simulink library "lib_FDM"  (R2019b)
settings: Solver=VariableStepAuto  StartTime=0.0  StopTime=10.0  RelTol=1e-3
values from neighbouring files (symbols this model uses):
  d = config.d_m    [computeTF.m]
undefined symbols (not defined in the file or in its folder): c_b_WGS, c_flat, c_grav, c_rot, c_rsma, Cd0, Cdcl, Cdcl2, Cl0, Cla, Cld, Cma, Cmd, Cmq, Cnb, Cnd, Cnr, Cra, Crd, Crp, Cy0, Cyb, Cyd, dmdt, Earth, HIL_Data, InitThrust, launchPos, me, mf, mp, Sref, tb, TF, theta0, WGS84
libraries: simulink_extras x14, $bdroot x7, simulink x5, lib_Fin_Deflections x3, aerolibasang x2, sharedtransform x1, aerolibtransform2 x1, aerolibbdyn x1, aerolibatmos2 x1, aerolibutil x1, aerolib6dof2 x1
(part 1 of 8)
settings Model: Creator=m.hiepp  LastModifiedBy=Guy
settings DataIOCC: ReturnWorkspaceOutputs=off
settings DebuggingCC: ArithmeticOperatorsInVariantConditions=warning
settings SFSimCC: CustomCodeUndefinedFunction=UseInterfaceOnly

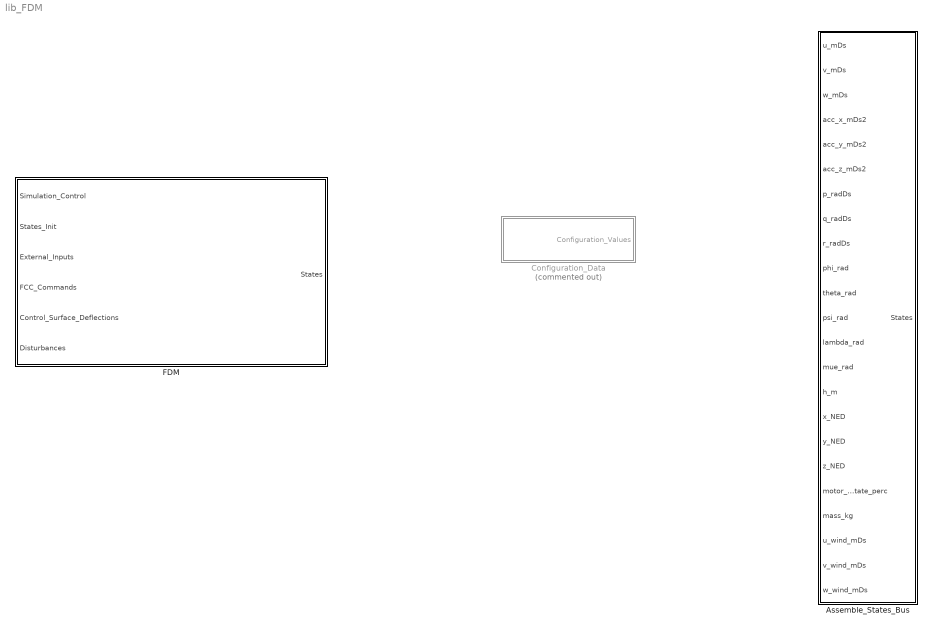
== system lib_FDM ==
  Assemble_States_Bus : Subsystem
  Configuration_Data : Subsystem  Commented=on
  FDM : Subsystem  Variant=on

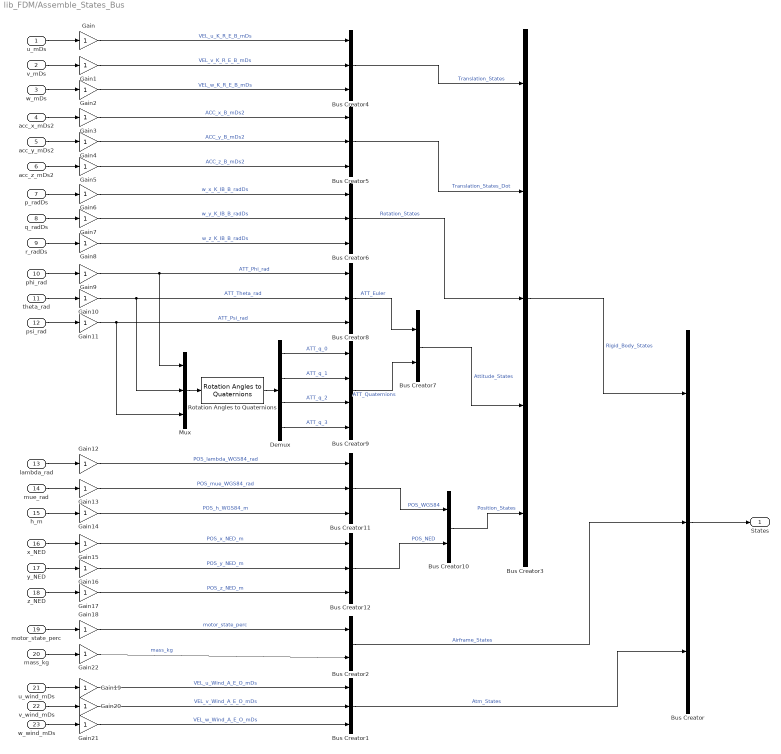
== system lib_FDM/Assemble_States_Bus ==
  u_mDs : Inport
  v_mDs : Inport  Port=2
  w_mDs : Inport  Port=3
  acc_x_mDs2 : Inport  Port=4
  acc_y_mDs2 : Inport  Port=5
  acc_z_mDs2 : Inport  Port=6
  p_radDs : Inport  Port=7
  q_radDs : Inport  Port=8
  r_radDs : Inport  Port=9
  phi_rad : Inport  Port=10
  theta_rad : Inport  Port=11
  psi_rad : Inport  Port=12
  lambda_rad : Inport  Port=13
  mue_rad : Inport  Port=14
  h_m : Inport  Port=15
  x_NED : Inport  Port=16
  y_NED : Inport  Port=17
  z_NED : Inport  Port=18
  motor_state_perc : Inport  Port=19
  mass_kg : Inport  Port=20
  u_wind_mDs : Inport  Port=21
  v_wind_mDs : Inport  Port=22
  w_wind_mDs : Inport  Port=23
  Bus Creator : BusCreator  Inputs=3  OutDataTypeStr=Bus: States_Bus
  Bus Creator1 : BusCreator  Inputs=3  OutDataTypeStr=Bus: Atm_States_Bus
  Bus Creator10 : BusCreator  Inputs=2  OutDataTypeStr=Bus: Position_States_Bus
  Bus Creator11 : BusCreator  Inputs=3  OutDataTypeStr=Bus: POS_WGS84_Bus
  Bus Creator12 : BusCreator  Inputs=3  OutDataTypeStr=Bus: POS_NED_Bus
  Bus Creator2 : BusCreator  Inputs=2  OutDataTypeStr=Bus: Airframe_States_Bus
  Bus Creator3 : BusCreator  Inputs=5  OutDataTypeStr=Bus: Rigid_Body_States_Bus
  Bus Creator4 : BusCreator  Inputs=3  OutDataTypeStr=Bus: Translation_States_Bus
  Bus Creator5 : BusCreator  Inputs=3  OutDataTypeStr=Bus: Translation_States_Dot_Bus
  Bus Creator6 : BusCreator  Inputs=3  OutDataTypeStr=Bus: Rotation_States_Bus
  Bus Creator7 : BusCreator  Inputs=2  OutDataTypeStr=Bus: Attitude_States_Bus
  Bus Creator8 : BusCreator  Inputs=3  OutDataTypeStr=Bus: ATT_Euler_Bus
  Bus Creator9 : BusCreator  Inputs=4  OutDataTypeStr=Bus: ATT_Quaternions_Bus
  Demux : Demux
  Gain{,1..22} (23 alike) : Gain
  Mux : Mux  Inputs=3
  Rotation Angles to Quaternions : sharedtransform/Rotation Angles to Quaternions  rotationOrder=ZYX  aMode=aMode
      settings: SourceProductName=Aerospace Blockset  SourceProductBaseCode=AE
  States : Outport  OutDataTypeStr=Bus: States_Bus  VectorParamsAs1DForOutWhenUnconnected=off
  wires:
  Bus Creator7/1 -> Bus Creator3/4  "Attitude_States"
  Mux/1 -> Rotation Angles to Quaternions/1
  Demux/3 -> Bus Creator9/3  "ATT_q_2"
  Demux/4 -> Bus Creator9/4  "ATT_q_3"
  Demux/1 -> Bus Creator9/1  "ATT_q_0"
  Bus Creator11/1 -> Bus Creator10/1  "POS_WGS84"
  w_mDs/1 -> Gain2/1
  Bus Creator1/1 -> Bus Creator/3  "Atm_States"
  Bus Creator9/1 -> Bus Creator7/2  "ATT_Quaternions"
  acc_x_mDs2/1 -> Gain3/1
  Bus Creator12/1 -> Bus Creator10/2  "POS_NED"
  Demux/2 -> Bus Creator9/2  "ATT_q_1"
  Bus Creator10/1 -> Bus Creator3/5  "Position_States"
  acc_z_mDs2/1 -> Gain5/1
  phi_rad/1 -> Gain9/1
  z_NED/1 -> Gain17/1
  Bus Creator2/1 -> Bus Creator/2  "Airframe_States"
  Bus Creator8/1 -> Bus Creator7/1  "ATT_Euler"
  w_wind_mDs/1 -> Gain21/1
  Bus Creator3/1 -> Bus Creator/1  "Rigid_Body_States"
  u_wind_mDs/1 -> Gain19/1
  Bus Creator4/1 -> Bus Creator3/1  "Translation_States"
  mue_rad/1 -> Gain13/1
  y_NED/1 -> Gain16/1
  Bus Creator6/1 -> Bus Creator3/3  "Rotation_States"
  Bus Creator5/1 -> Bus Creator3/2  "Translation_States_Dot"
  Rotation Angles to Quaternions/1 -> Demux/1
  x_NED/1 -> Gain15/1
  Bus Creator/1 -> States/1
  h_m/1 -> Gain14/1
  u_mDs/1 -> Gain/1
  lambda_rad/1 -> Gain12/1
  v_mDs/1 -> Gain1/1
  v_wind_mDs/1 -> Gain20/1
  motor_state_perc/1 -> Gain18/1
  psi_rad/1 -> Gain11/1
  theta_rad/1 -> Gain10/1
  r_radDs/1 -> Gain8/1
  p_radDs/1 -> Gain6/1
  q_radDs/1 -> Gain7/1
  acc_y_mDs2/1 -> Gain4/1
  Gain20/1 -> Bus Creator1/2  "VEL_v_Wind_A_E_O_mDs"
  Gain21/1 -> Bus Creator1/3  "VEL_w_Wind_A_E_O_mDs"
  Gain19/1 -> Bus Creator1/1  "VEL_u_Wind_A_E_O_mDs"
  Gain18/1 -> Bus Creator2/1  "motor_state_perc"
  Gain17/1 -> Bus Creator12/3  "POS_z_NED_m"
  Gain16/1 -> Bus Creator12/2  "POS_y_NED_m"
  Gain15/1 -> Bus Creator12/1  "POS_x_NED_m"
  Gain14/1 -> Bus Creator11/3  "POS_h_WGS84_m"
  Gain13/1 -> Bus Creator11/2  "POS_mue_WGS84_rad"
  Gain12/1 -> Bus Creator11/1  "POS_lambda_WGS84_rad"
  Gain11/1 -> Bus Creator8/3, Mux/3  "ATT_Psi_rad"
  Gain10/1 -> Bus Creator8/2, Mux/2  "ATT_Theta_rad"
  Gain9/1 -> Bus Creator8/1, Mux/1  "ATT_Phi_rad"
  Gain8/1 -> Bus Creator6/3  "w_z_K_IB_B_radDs"
  Gain7/1 -> Bus Creator6/2  "w_y_K_IB_B_radDs"
  Gain6/1 -> Bus Creator6/1  "w_x_K_IB_B_radDs"
  Gain5/1 -> Bus Creator5/3  "ACC_z_B_mDs2"
  Gain4/1 -> Bus Creator5/2  "ACC_y_B_mDs2"
  Gain3/1 -> Bus Creator5/1  "ACC_x_B_mDs2"
  Gain2/1 -> Bus Creator4/3  "VEL_w_K_R_E_B_mDs"
  Gain1/1 -> Bus Creator4/2  "VEL_v_K_R_E_B_mDs"
  Gain/1 -> Bus Creator4/1  "VEL_u_K_R_E_B_mDs"
  Gain22/1 -> Bus Creator2/2  "mass_kg"
  mass_kg/1 -> Gain22/1

== system lib_FDM/Configuration_Data ==
  Bus Creator : BusCreator  Inputs=10  OutDataTypeStr=Bus: Configuration_Values_Bus
  Constant : Constant  Value=HIL_Data.Configuration_Data.param1
  Configuration_Values : Outport  OutDataTypeStr=Bus: Configuration_Values_Bus  VectorParamsAs1DForOutWhenUnconnected=off
  wires:
  Constant/1 -> Bus Creator/1  "param1"
  Bus Creator/1 -> Configuration_Values/1

== system lib_FDM/FDM ==
  Simulation_Control : Inport  OutDataTypeStr=Bus: Simulation_Ctrl_Bus
  States_Init : Inport  Port=2  OutDataTypeStr=Bus: States_Bus
  External_Inputs : Inport  Port=3  OutDataTypeStr=Bus: External_Inputs_Bus
  FCC_Commands : Inport  Port=4  OutDataTypeStr=Bus: FCC_Commands_Bus
  Control_Surface_Deflections : Inport  Port=5  OutDataTypeStr=Bus: Control_Surface_Deflections_Bus
  Disturbances : Inport  Port=6  OutDataTypeStr=Bus: Disturbances_Bus
  FDM_Basic : Subsystem  VariantControl=VSS_FDM_BASIC  mask{FDM=HIL_Data.FDM, Basic=HIL_Data.FDM.Basic}
      mask prompts: FDM "FDM Data"; Basic "FDM Basic Data"
  FDM_Linear : Subsystem  VariantControl=VSS_FDM_LIN  mask{FDM=HIL_Data.FDM, Lin=HIL_Data.FDM.Lin, TF=HIL_Data.FDM.Lin.TF}
      mask prompts: FDM "FDM Data"; Lin "FDM Lin Data"; TF "Transfer Functions"
  FDM_Sophisticated : Subsystem  VariantControl=VSS_FDM_SOPH
  FDM_Student : Subsystem  VariantControl=VSS_FDM_STUD
  States : Outport  OutDataTypeStr=Bus: States_Bus  VectorParamsAs1DForOutWhenUnconnected=off

== system lib_FDM/FDM/FDM_Basic ==
  note: further commands??
  Simulation_Control : Inport  OutDataTypeStr=Bus: Simulation_Ctrl_Bus
  States_Init : Inport  Port=2  OutDataTypeStr=Bus: States_Bus
  External_Inputs : Inport  Port=3  OutDataTypeStr=Bus: External_Inputs_Bus
  FCC_Commands : Inport  Port=4  OutDataTypeStr=Bus: FCC_Commands_Bus
  Control_Surface_Deflections : Inport  Port=5  OutDataTypeStr=Bus: Control_Surface_Deflections_Bus
  Disturbances : Inport  Port=6  OutDataTypeStr=Bus: FCC_Commands_Bus
  Assemble_States_Bus : $bdroot/Assemble_States_Bus  SystemSampleTime=-1  Latency=0  AutoFrameSizeCalculation=off
  Bus Selector : BusSelector  OutputSignals=Translation_States.VEL_u_K_R_E_B_mDs,Translation_States.VEL_v_K_R_E_B_mDs,Translation_States.VEL_w_K_R_E_B_mDs
  Bus Selector1 : BusSelector  OutputSignals=Translation_States_Dot.ACC_x_B_mDs2,Translation_States_Dot.ACC_y_B_mDs2,Translation_States_Dot.ACC_z_B_mDs2
  Bus Selector2 : BusSelector  OutputSignals=Attitude_States.ATT_Phi_rad,Attitude_States.ATT_Theta_rad,Attitude_States.ATT_Psi_rad,Position_States.POS_WGS84.POS_lambda_ WGS84_rad,Position_States.POS_WGS84.POS_mue_ WGS84_rad,Position_States.POS_WGS84.POS_h_ WGS84_m,Position_States.POS_NED.POS_x_NED_m,Position_States.POS_NED.POS_y_NED_m,Position_States.POS_NED.POS_z_NED_m,Airframe_States.motor_state_perc,Airframe_States.mass_kg
  Bus Selector3 : BusSelector  OutputSignals=p_B_radDs,q_B_radDs,r_B_radDs
  Configuration_Data : $bdroot/Configuration_Data  Commented=on  SystemSampleTime=-1  Latency=0  AutoFrameSizeCalculation=off
  Constant : Constant  Value=-1
  Constant1 : Constant  Value=-1
  Constant2 : Constant  Value=-1
  Flight_State : Subsystem
  Motion_Kinematics : Subsystem
  State_Integration : Subsystem
  Terminator{,1,4..8} (7 alike) : Terminator
  States : Outport  OutDataTypeStr=Bus: States_Bus  VectorParamsAs1DForOutWhenUnconnected=off
  wires:
  Assemble_States_Bus/1 -> States/1
  FCC_Commands/1 -> Terminator/1
  Flight_State/1(vel_mDs) -> Terminator4/1
  Flight_State/4(mach) -> Terminator7/1
  Flight_State/5(q_kgDms2) -> Terminator8/1
  Flight_State/3(rho_kgDm3) -> Terminator6/1
  Flight_State/2(altitude_m) -> Terminator5/1
  State_Integration/1("FDM_States ") -> Motion_Kinematics/4(FDM_States)
  Motion_Kinematics/3(FDM_States_Dot) -> Bus Selector1/1, State_Integration/1(FDM_States_Dot)
  External_Inputs/1 -> Motion_Kinematics/2(External_Inputs)
  Simulation_Control/1 -> Motion_Kinematics/1(Simulation_Control), State_Integration/2(Simulation_Control)
  Control_Surface_Deflections/1 -> Motion_Kinematics/3(Control_Surface_Deflections)
  States_Init/1 -> State_Integration/3(States_Init)
  Motion_Kinematics/1(FDM_states) -> Bus Selector/1, Bus Selector2/1
  Bus Selector1/3 -> Assemble_States_Bus/6  "<ACC_z_B_mDs2>"
  Bus Selector1/2 -> Assemble_States_Bus/5  "<ACC_y_B_mDs2>"
  Bus Selector1/1 -> Assemble_States_Bus/4  "<ACC_x_B_mDs2>"
  Bus Selector/1 -> Assemble_States_Bus/1  "<VEL_u_K_R_E_B_mDs>"
  Bus Selector/2 -> Assemble_States_Bus/2  "<VEL_v_K_R_E_B_mDs>"
  Bus Selector/3 -> Assemble_States_Bus/3  "<VEL_w_K_R_E_B_mDs>"
  Bus Selector2/1 -> Assemble_States_Bus/10  "<ATT_Phi_rad>"
  Bus Selector2/2 -> Assemble_States_Bus/11  "<ATT_Theta_rad>"
  Bus Selector2/3 -> Assemble_States_Bus/12  "<ATT_Psi_rad>"
  Bus Selector2/4 -> Assemble_States_Bus/13  "<POS_lambda_ WGS84_rad>"
  Bus Selector2/5 -> Assemble_States_Bus/14  "<POS_mue_ WGS84_rad>"
  Bus Selector2/6 -> Assemble_States_Bus/15  "<POS_h_ WGS84_m>"
  Bus Selector2/7 -> Assemble_States_Bus/16  "<POS_x_NED_m>"
  Bus Selector2/8 -> Assemble_States_Bus/17  "<POS_y_NED_m>"
  Bus Selector2/9 -> Assemble_States_Bus/18  "<POS_z_NED_m>"
  Bus Selector2/10 -> Assemble_States_Bus/19  "<motor_state_perc>"
  Bus Selector2/11 -> Assemble_States_Bus/20  "<mass_kg>"
  Constant/1 -> Assemble_States_Bus/23
  Constant2/1 -> Assemble_States_Bus/21
  Constant1/1 -> Assemble_States_Bus/22
  Motion_Kinematics/2(FDM_Rot_Body) -> Bus Selector3/1
  Bus Selector3/1 -> Assemble_States_Bus/7  "<p_B_radDs>"
  Bus Selector3/2 -> Assemble_States_Bus/8  "<q_B_radDs>"
  Bus Selector3/3 -> Assemble_States_Bus/9  "<r_B_radDs>"
  Disturbances/1 -> Terminator1/1

== system lib_FDM/FDM/FDM_Linear ==
  note: further commands??
  Simulation_Control : Inport  OutDataTypeStr=Bus: Simulation_Ctrl_Bus
  States_Init : Inport  Port=2  OutDataTypeStr=Bus: States_Bus
  External_Inputs : Inport  Port=3  OutDataTypeStr=Bus: External_Inputs_Bus
  FCC_Commands : Inport  Port=4  OutDataTypeStr=Bus: FCC_Commands_Bus
  Control_Surface_Deflections : Inport  Port=5  OutDataTypeStr=Bus: Control_Surface_Deflections_Bus
  Disturbances : Inport  Port=6  OutDataTypeStr=Bus: FCC_Commands_Bus
  Assemble_States_Bus : $bdroot/Assemble_States_Bus  SystemSampleTime=-1  Latency=0  AutoFrameSizeCalculation=off
  Bus Selector : BusSelector  OutputSignals=Translation_States.VEL_u_K_R_E_B_mDs,Translation_States.VEL_v_K_R_E_B_mDs,Translation_States.VEL_w_K_R_E_B_mDs
  Bus Selector1 : BusSelector  OutputSignals=Translation_States_Dot.ACC_x_B_mDs2,Translation_States_Dot.ACC_y_B_mDs2,Translation_States_Dot.ACC_z_B_mDs2
  Bus Selector2 : BusSelector  OutputSignals=Attitude_States.ATT_Phi_rad,Attitude_States.ATT_Theta_rad,Attitude_States.ATT_Psi_rad,Position_States.POS_WGS84.POS_lambda_ WGS84_rad,Position_States.POS_WGS84.POS_mue_ WGS84_rad,Position_States.POS_WGS84.POS_h_ WGS84_m,Position_States.POS_NED.POS_x_NED_m,Position_States.POS_NED.POS_y_NED_m,Position_States.POS_NED.POS_z_NED_m,Airframe_States.motor_state_perc,Airframe_States.mass_kg
  Bus Selector3 : BusSelector  OutputSignals=p_B_radDs,q_B_radDs,r_B_radDs
  Configuration_Data : $bdroot/Configuration_Data  Commented=on  SystemSampleTime=-1  Latency=0  AutoFrameSizeCalculation=off
  Constant : Constant  Value=-1
  Constant1 : Constant  Value=-1
  Constant2 : Constant  Value=-1
  Flight_State : Subsystem
  Motion_Kinematics : Subsystem
  State_Integration : Subsystem
  Terminator{,1,4..8} (7 alike) : Terminator
  States : Outport  OutDataTypeStr=Bus: States_Bus  VectorParamsAs1DForOutWhenUnconnected=off
  wires:
  Assemble_States_Bus/1 -> States/1
  FCC_Commands/1 -> Terminator/1
  Flight_State/1(vel_mDs) -> Terminator4/1
  Flight_State/4(mach) -> Terminator7/1
  Flight_State/5(q_kgDms2) -> Terminator8/1
  Flight_State/3(rho_kgDm3) -> Terminator6/1
  Flight_State/2(altitude_m) -> Terminator5/1
  State_Integration/1("FDM_States ") -> Motion_Kinematics/4(FDM_States)
  Motion_Kinematics/3(FDM_States_Dot) -> Bus Selector1/1, State_Integration/1(FDM_States_Dot)
  External_Inputs/1 -> Motion_Kinematics/2(External_Inputs)
  Simulation_Control/1 -> Motion_Kinematics/1(Simulation_Control), State_Integration/2(Simulation_Control)
  Control_Surface_Deflections/1 -> Motion_Kinematics/3(Control_Surface_Deflections)
  States_Init/1 -> State_Integration/3(States_Init)
  Motion_Kinematics/1(FDM_states) -> Bus Selector/1, Bus Selector2/1
  Bus Selector1/3 -> Assemble_States_Bus/6  "<ACC_z_B_mDs2>"
  Bus Selector1/2 -> Assemble_States_Bus/5  "<ACC_y_B_mDs2>"
  Bus Selector1/1 -> Assemble_States_Bus/4  "<ACC_x_B_mDs2>"
  Bus Selector/1 -> Assemble_States_Bus/1  "<VEL_u_K_R_E_B_mDs>"
  Bus Selector/2 -> Assemble_States_Bus/2  "<VEL_v_K_R_E_B_mDs>"
  Bus Selector/3 -> Assemble_States_Bus/3  "<VEL_w_K_R_E_B_mDs>"
  Bus Selector2/1 -> Assemble_States_Bus/10  "<ATT_Phi_rad>"
  Bus Selector2/2 -> Assemble_States_Bus/11  "<ATT_Theta_rad>"
  Bus Selector2/3 -> Assemble_States_Bus/12  "<ATT_Psi_rad>"
  Bus Selector2/4 -> Assemble_States_Bus/13  "<POS_lambda_ WGS84_rad>"
  Bus Selector2/5 -> Assemble_States_Bus/14  "<POS_mue_ WGS84_rad>"
  Bus Selector2/6 -> Assemble_States_Bus/15  "<POS_h_ WGS84_m>"
  Bus Selector2/7 -> Assemble_States_Bus/16  "<POS_x_NED_m>"
  Bus Selector2/8 -> Assemble_States_Bus/17  "<POS_y_NED_m>"
  Bus Selector2/9 -> Assemble_States_Bus/18  "<POS_z_NED_m>"
  Bus Selector2/10 -> Assemble_States_Bus/19  "<motor_state_perc>"
  Bus Selector2/11 -> Assemble_States_Bus/20  "<mass_kg>"
  Constant/1 -> Assemble_States_Bus/23
  Constant2/1 -> Assemble_States_Bus/21
  Constant1/1 -> Assemble_States_Bus/22
  Motion_Kinematics/2(FDM_Rot_Body) -> Bus Selector3/1
  Bus Selector3/1 -> Assemble_States_Bus/7  "<p_B_radDs>"
  Bus Selector3/2 -> Assemble_States_Bus/8  "<q_B_radDs>"
  Bus Selector3/3 -> Assemble_States_Bus/9  "<r_B_radDs>"
  Disturbances/1 -> Terminator1/1

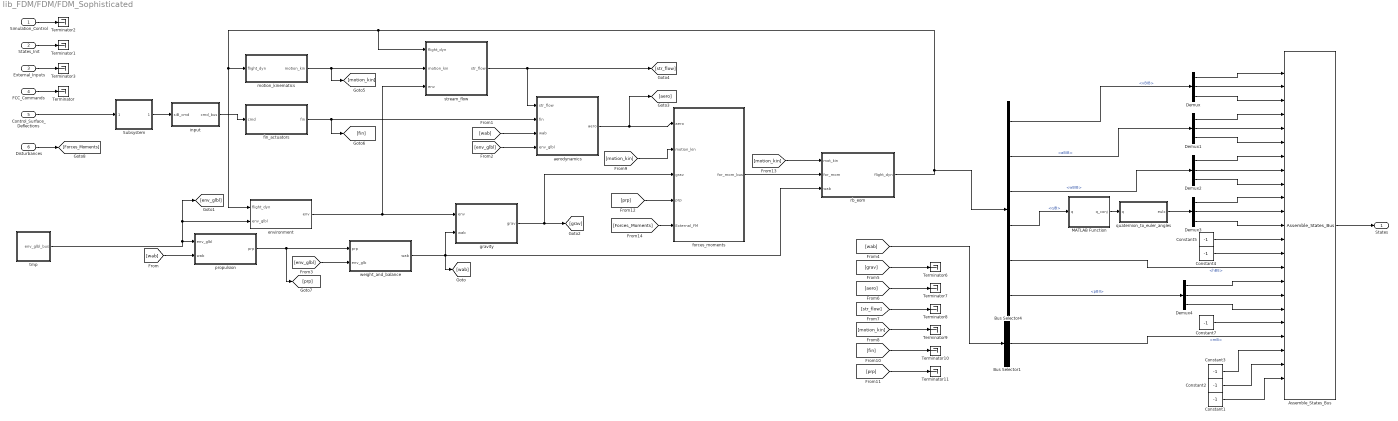
== system lib_FDM/FDM/FDM_Sophisticated ==
  Simulation_Control : Inport  OutDataTypeStr=Bus: Simulation_Ctrl_Bus
  States_Init : Inport  Port=2  OutDataTypeStr=Bus: States_Bus
  External_Inputs : Inport  Port=3  OutDataTypeStr=Bus: External_Inputs_Bus
  FCC_Commands : Inport  Port=4  OutDataTypeStr=Bus: FCC_Commands_Bus
  Control_Surface_Deflections : Inport  Port=5  OutDataTypeStr=Bus: Control_Surface_Deflections_Bus
  Disturbances : Inport  Port=6
  Assemble_States_Bus : $bdroot/Assemble_States_Bus  SystemSampleTime=-1  Latency=0  AutoFrameSizeCalculation=off
  Bus Selector1 : BusSelector  OutputSignals=mB
  Bus Selector4 : BusSelector  OutputSignals=vBIB,aBIB,wBIB,qIB,hBE,pBII
  Constant{1..5,7} (6 alike) : Constant  Value=-1
  Demux{,1..4} (5 alike) : Demux  Outputs=3
  MATLAB Function : MATLAB Function  TreatAsAtomicUnit=on
  Subsystem : Subsystem
  Terminator{,1..3,6..11} (10 alike) : Terminator
  aerodynamics : Subsystem
  environment : Subsystem
  fin_actuators : Subsystem
  forces_moments : Subsystem
  gravity : Subsystem
  input : Subsystem
  motion_kinematics : Subsystem
  propulsion : Subsystem
  quaternion_to_euler_angles : Subsystem
      mask help: transforms quaternions to Euler angles (roll, pitch, yaw)
      mask Help:
      | Name:
      | 
      |     quaternion_to_euler_angles
      | 
      | Description:
      | 
      |     This block implements the transformation of a quaternion into the
      |     corresponding Euler angles (zyx-sequence, roll, pitch, yaw).
      | 
      | Inputs  [size] [data type] [unit]:
      | 
      |     quaternion  [4] [double] [-]
      | 
      | Outputs  [size] [data type] [unit]:
      | 
      |     roll angle phi  [1] [double] [rad]
      |     pitch angle theta  [1] [double] [rad]
      |     yaw angle psi  [1] [double] [rad]
      mask Display:
      | %disp (' q --> (Phi,Theta,Psi) [rad]')
      | disp('q \rightarrow eu(\Phi;\Theta;\Psi)','texmode','on')
  rb_eom : Subsystem
  stream_flow : Subsystem
  tmp : Subsystem
  weight_and_balance : Subsystem
  States : Outport  OutDataTypeStr=Bus: States_Bus  VectorParamsAs1DForOutWhenUnconnected=off
  wires:
  environment/1(env) -> stream_flow/3(env), gravity/1(env)
  motion_kinematics/1(motion_kin) -> [motion_kin], stream_flow/2(motion_kin)
  [wab] -> aerodynamics/3(wab)
  [env_glbl] -> weight_and_balance/2(env_glb)
  fin_actuators/1(fin) -> aerodynamics/2(fin), [fin]
  propulsion/1(prp) -> [prp], weight_and_balance/1(prp)
  forces_moments/1(for_mom_bus) -> rb_eom/2(for_mom)
  aerodynamics/1(aero) -> [aero], forces_moments/1(aero)
  tmp/1(env_glbl_bus) -> environment/2(env_glbl), [env_glbl], propulsion/1(env_glbl)
  [aero] -> Terminator7/1
  [motion_kin] -> forces_moments/2(motion_kin)
  [motion_kin] -> Terminator9/1
  gravity/1(grav) -> forces_moments/3(grav), [grav]
  [motion_kin] -> rb_eom/1(mot_kin)
  [fin] -> Terminator10/1
  [str_flow] -> Terminator8/1
  [wab] -> Bus Selector1/1
  stream_flow/1(str_flow) -> [str_flow], aerodynamics/1(str_flow)
  weight_and_balance/1(wab) -> gravity/2(wab), rb_eom/3(wab), [wab]
  rb_eom/1(flight_dyn) -> motion_kinematics/1(flight_dyn), environment/1(flight_dyn), stream_flow/1(flight_dyn), Bus Selector4/1
  [env_glbl] -> aerodynamics/4(env_glbl)
  input/1(cmd_bus) -> fin_actuators/1(cmd)
  [prp] -> Terminator11/1
  [grav] -> Terminator6/1
  [prp] -> forces_moments/4(prp)
  [wab] -> propulsion/2(wab)
  FCC_Commands/1 -> Terminator/1
  States_Init/1 -> Terminator1/1
  Simulation_Control/1 -> Terminator2/1
  Demux2/1 -> Assemble_States_Bus/7
  Demux2/3 -> Assemble_States_Bus/9
  Demux2/2 -> Assemble_States_Bus/8
  Demux4/3 -> Assemble_States_Bus/18
  Demux4/1 -> Assemble_States_Bus/16
  Constant2/1 -> Assemble_States_Bus/22
  Assemble_States_Bus/1 -> States/1
  Demux3/1 -> Assemble_States_Bus/10
  Constant1/1 -> Assemble_States_Bus/23
  Constant7/1 -> Assemble_States_Bus/19
  Constant4/1 -> Assemble_States_Bus/14
  Constant5/1 -> Assemble_States_Bus/13
  Demux/2 -> Assemble_States_Bus/2
  Demux3/3 -> Assemble_States_Bus/12
  Demux1/1 -> Assemble_States_Bus/4
  Demux/1 -> Assemble_States_Bus/1
  Demux/3 -> Assemble_States_Bus/3
  Constant3/1 -> Assemble_States_Bus/21
  Demux1/2 -> Assemble_States_Bus/5
  Demux1/3 -> Assemble_States_Bus/6
  Demux4/2 -> Assemble_States_Bus/17
  Bus Selector4/1 -> Demux/1  "<vBIB>"
  Bus Selector4/2 -> Demux1/1  "<aBIB>"
  Bus Selector4/3 -> Demux2/1  "<wBIB>"
  Bus Selector4/4 -> MATLAB Function/1(q)  "<qIB>"
  MATLAB Function/1(q_conj) -> quaternion_to_euler_angles/1(q)
  quaternion_to_euler_angles/1(eulx) -> Demux3/1
  Demux3/2 -> Assemble_States_Bus/11
  Bus Selector4/6 -> Demux4/1  "<pBII>"
  Bus Selector4/5 -> Assemble_States_Bus/15  "<hBE>"
  External_Inputs/1 -> Terminator3/1
  [Forces_Moments] -> forces_moments/5(External_FM)
  Disturbances/1 -> [Forces_Moments]
  Bus Selector1/1 -> Assemble_States_Bus/20  "<mB>"
  Control_Surface_Deflections/1 -> Subsystem/1(Servo Deflections)
  Subsystem/1(siB_cmd) -> input/1(siB_cmd)

== system lib_FDM/FDM/FDM_Student ==
  note: TBD!
  note: TBD
  note: TBD: insert propulsion
  note: TBD!
  note: TBD!
  note: TBD!
  Simulation_Control : Inport  OutDataTypeStr=Bus: Simulation_Ctrl_Bus
  States_Init : Inport  Port=2  OutDataTypeStr=Bus: States_Bus
  External_Inputs : Inport  Port=3  OutDataTypeStr=Bus: External_Inputs_Bus
  FCC_Commands : Inport  Port=4  OutDataTypeStr=Bus: FCC_Commands_Bus
  Control_Surface_Deflections : Inport  Port=5  OutDataTypeStr=Bus: Control_Surface_Deflections_Bus
  Aerodynamics : Subsystem
  Assemble_States_Bus : $bdroot/Assemble_States_Bus  SystemSampleTime=-1  Latency=0  AutoFrameSizeCalculation=off
  Configuration_Data : $bdroot/Configuration_Data  Commented=on  SystemSampleTime=-1  Latency=0  AutoFrameSizeCalculation=off
  Demux{,1..5} (6 alike) : Demux  Outputs=3
  Global Calculations : Subsystem
  MATLAB Function : MATLAB Function  TreatAsAtomicUnit=on
  MATLAB Function1 : MATLAB Function  TreatAsAtomicUnit=on
  Memory : Memory
  Reverse Fin Deflection : lib_Fin_Deflections/Reverse Fin Deflection  Control_Surfaces=HIL_Data.Control_Surfaces
  Selector : Selector  InputPortWidth=3  IndexOptions=Index vector (dialog)  Indices=[1]  OutputSizes=1
  Simple Variable Mass 6DOF ECEF (Quaternion) : aerolib6dof2/6DOF ECEF (Quaternion)  units=Metric (MKS)  mtype=Simple Variable  xg_0=[launchPos(1) launchPos(2) launchPos(3)]  Vm_0=[0 0 0]  eul_0=[0 theta0 0]  pm_0=[0 0 0]  mass_0=mf  mass_e=me  mass_f=mf  inertia=inertia  inertia_e=Ie  inertia_f=If  vre_flag=off  abi_flag=on  ptype=Earth (WGS84)  R=6378137  F=1/298.257223563  w_E=7292115e-11  angle_in=Internal  LG0=0  quat_statename=''  pm_statename=''  Vm_statename=''  posECEF_statename=''  posECI_statename=''  LG_statename=''  mass_statename=''
      settings: SourceProductName=Aerospace Blockset  SourceProductBaseCode=AE
  TBD : Constant  Value=-1
  TBD1 : Constant  Value=-1
  Terminator{,1..14} (15 alike) : Terminator
  Transpose : Math  Operator=transpose  SaturateOnIntegerOverflow=on
  States : Outport  OutDataTypeStr=Bus: States_Bus  VectorParamsAs1DForOutWhenUnconnected=off
  wires:
  Aerodynamics/2("[Mxb Myb Mzb]") -> Simple Variable Mass 6DOF ECEF (Quaternion)/2
  [dmdt] -> Simple Variable Mass 6DOF ECEF (Quaternion)/3
  Aerodynamics/1("[Fxb Fyb Fzb]") -> Simple Variable Mass 6DOF ECEF (Quaternion)/1
  Assemble_States_Bus/1 -> States/1
  Reverse Fin Deflection/1 -> Aerodynamics/3(delta R)  "delta_r"
  Reverse Fin Deflection/2 -> Aerodynamics/2(delta P)  "delta_p"
  Reverse Fin Deflection/3 -> Aerodynamics/1("delta Y ")  "delta_y"
  Control_Surface_Deflections/1 -> Reverse Fin Deflection/2
  Simple Variable Mass 6DOF ECEF (Quaternion)/1 -> MATLAB Function/2(VelECEF), Terminator/1
  Simple Variable Mass 6DOF ECEF (Quaternion)/2 -> Terminator1/1, MATLAB Function/3(PosECEF)
  Demux/1 -> Assemble_States_Bus/13
  Demux/2 -> Assemble_States_Bus/14
  Demux/3 -> Assemble_States_Bus/15
  Simple Variable Mass 6DOF ECEF (Quaternion)/3 -> Demux/1
  Demux1/3 -> Assemble_States_Bus/12
  Demux1/2 -> Assemble_States_Bus/11
  Demux1/1 -> Assemble_States_Bus/10
  Simple Variable Mass 6DOF ECEF (Quaternion)/4 -> Demux1/1, Selector/1
  Simple Variable Mass 6DOF ECEF (Quaternion)/5 -> Terminator2/1
  Simple Variable Mass 6DOF ECEF (Quaternion)/6 -> Transpose/1, Terminator3/1
  Simple Variable Mass 6DOF ECEF (Quaternion)/7 -> Terminator4/1, MATLAB Function/1(ECEF2NED)
  Demux2/1 -> Assemble_States_Bus/1
  Demux2/2 -> Assemble_States_Bus/2
  Demux2/3 -> Assemble_States_Bus/3
  Simple Variable Mass 6DOF ECEF (Quaternion)/8 -> Demux2/1
  Demux3/1 -> Assemble_States_Bus/7
  Demux3/2 -> Assemble_States_Bus/8
  Demux3/3 -> Assemble_States_Bus/9
  Simple Variable Mass 6DOF ECEF (Quaternion)/10 -> Demux3/1
  Simple Variable Mass 6DOF ECEF (Quaternion)/9 -> Terminator5/1
  Simple Variable Mass 6DOF ECEF (Quaternion)/11 -> Terminator6/1
  Demux4/1 -> Assemble_States_Bus/4
  Demux4/2 -> Assemble_States_Bus/5
  Demux4/3 -> Assemble_States_Bus/6
  Simple Variable Mass 6DOF ECEF (Quaternion)/12 -> Demux4/1
  Simple Variable Mass 6DOF ECEF (Quaternion)/14 -> MATLAB Function1/1(BodyAcc), Terminator7/1
  Simple Variable Mass 6DOF ECEF (Quaternion)/13 -> Terminator8/1
  Demux5/1 -> Assemble_States_Bus/16
  Demux5/2 -> Assemble_States_Bus/17
  Demux5/3 -> Assemble_States_Bus/18
  MATLAB Function/2(PosNED) -> Demux5/1
  MATLAB Function/1(VelNED) -> Terminator9/1
  TBD/1 -> Assemble_States_Bus/20, Assemble_States_Bus/19
  TBD1/1 -> Assemble_States_Bus/22, Assemble_States_Bus/23, Assemble_States_Bus/21
  Transpose/1 -> MATLAB Function1/2(BODY2NED)
  MATLAB Function1/1(NEDAcc) -> Terminator10/1
  Selector/1 -> Memory/1
  Memory/1 -> Reverse Fin Deflection/1
  Simulation_Control/1 -> Terminator11/1
  States_Init/1 -> Terminator12/1
  External_Inputs/1 -> Terminator13/1
  FCC_Commands/1 -> Terminator14/1

== system lib_FDM/FDM/FDM_Basic/Flight_State ==
  Constant : Constant  Commented=on  Value=Basic.FS.vel_mDs
  Constant1 : Constant  Commented=on  Value=Basic.FS.alt_m
  Constant2 : Constant  Commented=on  Value=Basic.FS.rho_kgDm3
  Constant3 : Constant  Commented=on  Value=Basic.FS.mach
  Constant4 : Constant  Commented=on  Value=Basic.FS.q_kgDms2
  Constant5 : Constant  Value=-1
  vel_mDs : Outport  VectorParamsAs1DForOutWhenUnconnected=off
  altitude_m : Outport  Port=2  VectorParamsAs1DForOutWhenUnconnected=off
  rho_kgDm3 : Outport  Port=3  VectorParamsAs1DForOutWhenUnconnected=off
  mach : Outport  Port=4  VectorParamsAs1DForOutWhenUnconnected=off
  q_kgDms2 : Outport  Port=5  VectorParamsAs1DForOutWhenUnconnected=off
  wires:
  Constant5/1 -> altitude_m/1, q_kgDms2/1, mach/1, rho_kgDm3/1, vel_mDs/1

== system lib_FDM/FDM/FDM_Basic/Motion_Kinematics ==
  note: Add Transfer Functions from fin deflection to aero angles!!!
  Simulation_Control : Inport  OutDataTypeStr=Bus: Simulation_Ctrl_Bus
  External_Inputs : Inport  Port=2  OutDataTypeStr=Bus: External_Inputs_Bus
  Control_Surface_Deflections : Inport  Port=3  OutDataTypeStr=Bus: Control_Surface_Deflections_Bus
  FDM_States : Inport  Port=4  OutDataTypeStr=Bus: FDM_States_Bus
  Add : Sum  Inputs=+++
  Add1 : Sum  Inputs=+++
  Add2 : Sum  Inputs=+++
  Bus Creator : BusCreator  Inputs=4  OutDataTypeStr=Bus: FDM_States_Dot_Bus
  Bus Creator1 : BusCreator  Inputs=3  OutDataTypeStr=Bus: ATT_Euler_Dot_Bus
  Bus Creator2 : BusCreator  Inputs=3  OutDataTypeStr=Bus: Translation_States_Dot_Bus
  Bus Creator3 : BusCreator  Inputs=3  OutDataTypeStr=Bus: POS_WGS84_Dot_Bus
  Bus Creator4 : BusCreator  Inputs=1  OutDataTypeStr=Bus: Airframe_States_Dot_Bus
  Bus Creator5 : BusCreator  Inputs=3  OutDataTypeStr=Bus: POS_NED_Dot_Bus
  Bus Creator6 : BusCreator  Inputs=2  OutDataTypeStr=Bus: Position_States_Dot_Bus
  Bus Creator7 : BusCreator  Inputs=3  OutDataTypeStr=Bus: FDM_Rot_Body_Bus
  Bus Selector : BusSelector  OutputSignals=Airframe_States.mass_kg
  Bus Selector1 : BusSelector  OutputSignals=FDM_External_Inputs.Motor_Ignition_flg
  Bus Selector10 : BusSelector  OutputSignals=FDM_Ctrl.enable_drag_flg
  Bus Selector2 : BusSelector  OutputSignals=FDM_Ctrl.enable_propulsion_flg
  Bus Selector3 : BusSelector  OutputSignals=Translation_States.VEL_u_K_R_E_B_mDs,Translation_States.VEL_v_K_R_E_B_mDs,Translation_States.VEL_w_K_R_E_B_mDs
  Bus Selector4 : BusSelector  OutputSignals=Attitude_States
  Bus Selector5 : BusSelector  OutputSignals=Attitude_States.ATT_Phi_rad
  Bus Selector6 : BusSelector  OutputSignals=Attitude_States
  Bus Selector7 : BusSelector  OutputSignals=Position_States.POS_WGS84.POS_mue_ WGS84_rad,Position_States.POS_WGS84.POS_h_ WGS84_m
  Bus Selector8 : BusSelector  OutputSignals=Attitude_States.ATT_Phi_rad,Attitude_States.ATT_Theta_rad,Attitude_States.ATT_Psi_rad
  Bus Selector9 : BusSelector  OutputSignals=FDM_Ctrl.enable_gravity_flg
  Constant3 : Constant  Value=-1
  Divide : Product  Inputs=*/
  Drag : Subsystem  TreatAsAtomicUnit=on
  Gravity : Subsystem  TreatAsAtomicUnit=on
  NED2PosWGS84Dot : Subsystem
  Propulsion : Subsystem
  Reverse Fin Deflection : lib_Fin_Deflections/Reverse Fin Deflection  Control_Surfaces=HIL_Data.Control_Surfaces
  dp2az : TransferFcn  Numerator=TF.dp2az.num  Denominator=TF.dp2az.denom
  dp2pitch : TransferFcn  Numerator=TF.dp2pitch.num  Denominator=TF.dp2pitch.denom
  dr2roll : TransferFcn  Numerator=TF.dr2roll.num  Denominator=TF.dr2roll.denom
  dy2ay : TransferFcn  Numerator=TF.dy2ay.num  Denominator=TF.dy2ay.denom
  dy2yaw : TransferFcn  Numerator=TF.dy2yaw.num  Denominator=TF.dy2yaw.denom
  pqr2EulerDot : Subsystem
  uvw2PosNEDDot : Subsystem
  FDM_states : Outport  OutDataTypeStr=Bus: FDM_States_Bus  VectorParamsAs1DForOutWhenUnconnected=off
  FDM_Rot_Body : Outport  Port=2  OutDataTypeStr=Bus: FDM_Rot_Body_Bus  VectorParamsAs1DForOutWhenUnconnected=off
  FDM_States_Dot : Outport  Port=3  OutDataTypeStr=Bus: FDM_States_Dot_Bus  VectorParamsAs1DForOutWhenUnconnected=off
  wires:
  Reverse Fin Deflection/3 -> dy2yaw/1, dy2ay/1  "delta_y"
  Bus Selector2/1 -> Propulsion/Enable  "<enable_propulsion_flg>"
  dr2roll/1 -> pqr2EulerDot/2(p), Bus Creator7/1  "p_B_radDs"
  dp2pitch/1 -> pqr2EulerDot/3(q), Bus Creator7/2  "q_B_radDs"
  Reverse Fin Deflection/2 -> dp2pitch/1, dp2az/1  "delta_p"
  Reverse Fin Deflection/1 -> dr2roll/1  "delta_r"
  dy2yaw/1 -> Bus Creator7/3, pqr2EulerDot/4(r)  "r_B_radDs"
  Propulsion/1(F_x_prop_N) -> Divide/1
  Bus Creator/1 -> FDM_States_Dot/1
  pqr2EulerDot/3(psi_dot) -> Bus Creator1/3  "ATT_Dot_Psi_radDs"
  pqr2EulerDot/2(theta_dot) -> Bus Creator1/2  "ATT_Dot_Theta_radDs"
  pqr2EulerDot/1(phi_dot) -> Bus Creator1/1  "ATT_Dot_Phi_radDs"
  Bus Creator1/1 -> Bus Creator/1  "ATT_Euler_Dot"
  Bus Creator2/1 -> Bus Creator/2  "Translation_States_Dot"
  dp2az/1 -> Add2/1
  dy2ay/1 -> Add1/1
  Divide/1 -> Add/1
  Add/1 -> Bus Creator2/1  "ACC_x_B_mDs2"
  Add1/1 -> Bus Creator2/2  "ACC_y_B_mDs2"
  Add2/1 -> Bus Creator2/3  "ACC_z_B_mDs2"
  NED2PosWGS84Dot/3(h_dot_mDs) -> Bus Creator3/3  "POS_h_Dot_WGS84_mDs"
  NED2PosWGS84Dot/2(mue_dot_radDs) -> Bus Creator3/2  "POS_mue_Dot_WGS84_radDs"
  NED2PosWGS84Dot/1(lambda_dot_radDs) -> Bus Creator3/1  "POS_lambda_Dot_WGS84_radDs"
  Bus Creator4/1 -> Bus Creator/4  "Airframe_States_Dot"
  Propulsion/2(motor_state_perc_dot) -> Bus Creator4/1  "Motor_state_dot_percDs"
  External_Inputs/1 -> Bus Selector1/1
  Simulation_Control/1 -> Bus Selector10/1, Bus Selector9/1, Bus Selector2/1
  Bus Selector1/1 -> Propulsion/1(Motor_Ignition_flg)  "<Motor_Ignition_flg>"
  Bus Selector4/1 -> pqr2EulerDot/1(ATT)  "<Attitude_States>"
  Bus Selector5/1 -> Reverse Fin Deflection/1  "<ATT_Phi_rad>"
  Control_Surface_Deflections/1 -> Reverse Fin Deflection/2
  Bus Selector/1 -> Divide/2  "<mass_kg>"
  Bus Selector3/1 -> uvw2PosNEDDot/1(u)  "<VEL_u_K_R_E_B_mDs>"
  Bus Selector3/2 -> uvw2PosNEDDot/2(v)  "<VEL_v_K_R_E_B_mDs>"
  Bus Selector3/3 -> uvw2PosNEDDot/3(w)  "<VEL_w_K_R_E_B_mDs>"
  uvw2PosNEDDot/1(x_dot_mDs) -> Bus Creator5/1, NED2PosWGS84Dot/3(x_dot_NED_mDs)  "POS_x_Dot_NED_mDs"
  uvw2PosNEDDot/2(y_dot_mDs) -> NED2PosWGS84Dot/4(y_dot_NED_mDs), Bus Creator5/2  "POS_y_Dot_NED_mDs"
  uvw2PosNEDDot/3(z_dot_mDs) -> NED2PosWGS84Dot/5(z_dot_NED_mDs), Bus Creator5/3  "POS_z_Dot_NED_mDs"
  Bus Creator6/1 -> Bus Creator/3  "Position_States_Dot"
  Bus Creator3/1 -> Bus Creator6/1  "POS_WGS84_Dot"
  Bus Creator5/1 -> Bus Creator6/2  "POS_NED_Dot"
  Bus Selector6/1 -> uvw2PosNEDDot/4(ATT)  "<Attitude_States>"
  Bus Selector7/1 -> NED2PosWGS84Dot/1(mue_rad)  "<POS_mue_ WGS84_rad>"
  Bus Selector7/2 -> NED2PosWGS84Dot/2(h_m)  "<POS_h_ WGS84_m>"
  Gravity/1(acc_x_grav_mDs) -> Add/2
  Constant3/1 -> Drag/2(beta), Drag/1(alpha)
  Gravity/2(acc_y_grav_mDs) -> Add1/2
  Gravity/3(acc_z_grav_mDs) -> Add2/2
  Bus Selector8/1 -> Gravity/1(phi)  "<ATT_Phi_rad>"
  Bus Selector8/2 -> Gravity/2(theta)  "<ATT_Theta_rad>"
  Bus Selector8/3 -> Gravity/3(psi)  "<ATT_Psi_rad>"
  Bus Selector9/1 -> Gravity/Enable  "<enable_gravity_flg>"
  Bus Selector10/1 -> Drag/Enable  "<enable_drag_flg>"
  Drag/1(acc_x_drag_mDs2) -> Add/3
  Drag/2(acc_y_drag_mDs2) -> Add1/3
  Drag/3(acc_z_drag_mDs2) -> Add2/3
  FDM_States/1 -> FDM_states/1, Bus Selector5/1, Bus Selector6/1, Bus Selector3/1, Bus Selector7/1, Bus Selector8/1, Bus Selector/1, Bus Selector4/1
  Bus Creator7/1 -> FDM_Rot_Body/1

== system lib_FDM/FDM/FDM_Basic/State_Integration ==
  FDM_States_Dot : Inport  OutDataTypeStr=Bus: FDM_States_Dot_Bus
  Simulation_Control : Inport  Port=2  OutDataTypeStr=Bus: Simulation_Ctrl_Bus
  States_Init : Inport  Port=3  OutDataTypeStr=Bus: States_Bus
  ATT_Integration : Subsystem
  Bus Creator : BusCreator  Inputs=4  OutDataTypeStr=Bus: FDM_States_Bus
  Bus Creator1 : BusCreator  Inputs=3  OutDataTypeStr=Bus: ATT_Euler_Bus
  Bus Creator2 : BusCreator  Inputs=3  OutDataTypeStr=Bus: Translation_States_Bus
  Bus Creator3 : BusCreator  Inputs=2  OutDataTypeStr=Bus: Airframe_States_Bus
  Bus Creator4 : BusCreator  Inputs=3  OutDataTypeStr=Bus: POS_WGS84_Bus
  Bus Creator5 : BusCreator  Inputs=3  OutDataTypeStr=Bus: POS_NED_Bus
  Bus Creator6 : BusCreator  Inputs=2  OutDataTypeStr=Bus: Position_States_Bus
  Bus Selector : BusSelector  OutputSignals=ATT_Euler_Dot.ATT_Dot_Phi_radDs,ATT_Euler_Dot.ATT_Dot_Theta_radDs,ATT_Euler_Dot.ATT_Dot_Psi_radDs
  Bus Selector1 : BusSelector  OutputSignals=Translation_States_Dot.ACC_x_B_mDs2,Translation_States_Dot.ACC_y_B_mDs2,Translation_States_Dot.ACC_z_B_mDs2
  Bus Selector2 : BusSelector  OutputSignals=Airframe_States_Dot.Motor_state_dot_percDs
  Bus Selector3 : BusSelector  OutputSignals=Position_States_Dot.POS_WGS84_Dot.POS_lambda_Dot_WGS84_radDs,Position_States_Dot.POS_WGS84_Dot.POS_mue_Dot_WGS84_radDs,Position_States_Dot.POS_WGS84_Dot.POS_h_Dot_WGS84_mDs
  Bus Selector4 : BusSelector  OutputSignals=Position_States_Dot.POS_NED_Dot.POS_x_Dot_NED_mDs,Position_States_Dot.POS_NED_Dot.POS_y_Dot_NED_mDs,Position_States_Dot.POS_NED_Dot.POS_z_Dot_NED_mDs
  Mass_Balance : Subsystem
  Motor_State_Integration : Subsystem
  POS_NED_Integrator : Subsystem
  POS_WGS84_Integrator : Subsystem
  Terminator1 : Terminator
  Terminator2 : Terminator
  Terminator3 : Terminator
  VEL_Integrator : Subsystem
  "FDM_States " : Outport  OutDataTypeStr=Bus: FDM_States_Bus  VectorParamsAs1DForOutWhenUnconnected=off
  wires:
  Mass_Balance/4(I_z_kgm2) -> Terminator3/1
  Mass_Balance/2(I_x_kgm2) -> Terminator1/1
  Mass_Balance/3(I_y_kgm2) -> Terminator2/1
  FDM_States_Dot/1 -> Bus Selector2/1, Bus Selector4/1, Bus Selector3/1, Bus Selector1/1, Bus Selector/1
  Bus Selector/1 -> ATT_Integration/3(phi_dot_radDs)  "<ATT_Dot_Phi_radDs>"
  Bus Selector/2 -> ATT_Integration/4(theta_dot_radDs)  "<ATT_Dot_Theta_radDs>"
  Bus Selector/3 -> ATT_Integration/5(psi_dot_radDs)  "<ATT_Dot_Psi_radDs>"
  Bus Creator/1 -> "FDM_States "/1
  ATT_Integration/3(psi_rad) -> Bus Creator1/3  "ATT_Psi_rad"
  ATT_Integration/2(theta_rad) -> Bus Creator1/2  "ATT_Theta_rad"
  ATT_Integration/1(phi_rad) -> Bus Creator1/1  "ATT_Phi_rad"
  Bus Creator1/1 -> Bus Creator/1  "Attitude_States"
  Simulation_Control/1 -> Motor_State_Integration/1(Simulation_Control), POS_NED_Integrator/1(Simulation_Control), POS_WGS84_Integrator/1(Simulation_Control), VEL_Integrator/1(Simulation_Control), ATT_Integration/1(Simulation_Control)
  States_Init/1 -> Motor_State_Integration/2(Initial_States), POS_NED_Integrator/2(Initial_States), POS_WGS84_Integrator/2(Initial_States), VEL_Integrator/2(Initial_States), ATT_Integration/2(Initial_States)
  Bus Creator2/1 -> Bus Creator/2  "Translation_States"
  VEL_Integrator/1(u_mDs) -> Bus Creator2/1  "VEL_u_K_R_E_B_mDs"
  VEL_Integrator/2(v_mDs) -> Bus Creator2/2  "VEL_v_K_R_E_B_mDs"
  VEL_Integrator/3(w_mDs) -> Bus Creator2/3  "VEL_w_K_R_E_B_mDs"
  Bus Selector1/3 -> VEL_Integrator/5(az_mDs2)  "<ACC_z_B_mDs2>"
  Bus Selector1/2 -> VEL_Integrator/4(ay_mDs2)  "<ACC_y_B_mDs2>"
  Bus Selector1/1 -> VEL_Integrator/3(ax_mDs2)  "<ACC_x_B_mDs2>"
  Bus Selector2/1 -> Motor_State_Integration/3(motor_state_dot_percDs)  "<Motor_state_dot_percDs>"
  Bus Creator3/1 -> Bus Creator/4  "Airframe_States"
  Motor_State_Integration/1(motor_state_perc) -> Mass_Balance/1(motor_state_perc), Bus Creator3/1  "motor_state_perc"
  Mass_Balance/1(mass_kg) -> Bus Creator3/2  "mass_kg"
  Bus Creator6/1 -> Bus Creator/3  "Position_States"
  Bus Creator4/1 -> Bus Creator6/1  "POS_WGS84"
  Bus Creator5/1 -> Bus Creator6/2  "POS_NED"
  POS_WGS84_Integrator/1(lambda_rad) -> Bus Creator4/1  "POS_lambda_ WGS84_rad"
  POS_WGS84_Integrator/2(mue_rad) -> Bus Creator4/2  "POS_mue_ WGS84_rad"
  POS_WGS84_Integrator/3(h_m) -> Bus Creator4/3  "POS_h_ WGS84_m"
  POS_NED_Integrator/1(x_m) -> Bus Creator5/1  "POS_x_NED_m"
  POS_NED_Integrator/2(y_m) -> Bus Creator5/2  "POS_y_NED_m"
  POS_NED_Integrator/3(z_m) -> Bus Creator5/3  "POS_z_NED_m"
  Bus Selector3/1 -> POS_WGS84_Integrator/3(lambda_dot_radDs)  "<POS_lambda_Dot_WGS84_radDs>"
  Bus Selector3/2 -> POS_WGS84_Integrator/4(mue_dot_radDs)  "<POS_mue_Dot_WGS84_radDs>"
  Bus Selector3/3 -> POS_WGS84_Integrator/5(h_dot_mDs)  "<POS_h_Dot_WGS84_mDs>"
  Bus Selector4/1 -> POS_NED_Integrator/3(x_dot_mDs)  "<POS_x_Dot_NED_mDs>"
  Bus Selector4/2 -> POS_NED_Integrator/4(y_dot_mDs)  "<POS_y_Dot_NED_mDs>"
  Bus Selector4/3 -> POS_NED_Integrator/5(z_dot_mDs)  "<POS_z_Dot_NED_mDs>"

== system lib_FDM/FDM/FDM_Linear/Flight_State ==
  Constant : Constant  Value=Lin.FS.vel_mDs
  Constant1 : Constant  Value=Lin.FS.alt_m
  Constant2 : Constant  Value=Lin.FS.rho_kgDm3
  Constant3 : Constant  Value=Lin.FS.mach
  Constant4 : Constant  Value=Lin.FS.q_kgDms2
  vel_mDs : Outport  VectorParamsAs1DForOutWhenUnconnected=off
  altitude_m : Outport  Port=2  VectorParamsAs1DForOutWhenUnconnected=off
  rho_kgDm3 : Outport  Port=3  VectorParamsAs1DForOutWhenUnconnected=off
  mach : Outport  Port=4  VectorParamsAs1DForOutWhenUnconnected=off
  q_kgDms2 : Outport  Port=5  VectorParamsAs1DForOutWhenUnconnected=off
  wires:
  Constant/1 -> vel_mDs/1
  Constant1/1 -> altitude_m/1
  Constant4/1 -> q_kgDms2/1
  Constant3/1 -> mach/1
  Constant2/1 -> rho_kgDm3/1

== system lib_FDM/FDM/FDM_Linear/Motion_Kinematics ==
  note: Add Transfer Functions from fin deflection to aero angles!!!
  Simulation_Control : Inport  OutDataTypeStr=Bus: Simulation_Ctrl_Bus
  External_Inputs : Inport  Port=2  OutDataTypeStr=Bus: External_Inputs_Bus
  Control_Surface_Deflections : Inport  Port=3  OutDataTypeStr=Bus: Control_Surface_Deflections_Bus
  FDM_States : Inport  Port=4  OutDataTypeStr=Bus: FDM_States_Bus
  Add : Sum  Inputs=+++
  Add1 : Sum  Inputs=+++
  Add2 : Sum  Inputs=+++
  Bus Creator : BusCreator  Inputs=4  OutDataTypeStr=Bus: FDM_States_Dot_Bus
  Bus Creator1 : BusCreator  Inputs=3  OutDataTypeStr=Bus: ATT_Euler_Dot_Bus
  Bus Creator2 : BusCreator  Inputs=3  OutDataTypeStr=Bus: Translation_States_Dot_Bus
  Bus Creator3 : BusCreator  Inputs=3  OutDataTypeStr=Bus: POS_WGS84_Dot_Bus
  Bus Creator4 : BusCreator  Inputs=1  OutDataTypeStr=Bus: Airframe_States_Dot_Bus
  Bus Creator5 : BusCreator  Inputs=3  OutDataTypeStr=Bus: POS_NED_Dot_Bus
  Bus Creator6 : BusCreator  Inputs=2  OutDataTypeStr=Bus: Position_States_Dot_Bus
  Bus Creator7 : BusCreator  Inputs=3  OutDataTypeStr=Bus: FDM_Rot_Body_Bus
  Bus Selector : BusSelector  OutputSignals=Airframe_States.mass_kg
  Bus Selector1 : BusSelector  OutputSignals=FDM_External_Inputs.Motor_Ignition_flg
  Bus Selector10 : BusSelector  OutputSignals=FDM_Ctrl.enable_drag_flg
  Bus Selector2 : BusSelector  OutputSignals=FDM_Ctrl.enable_propulsion_flg
  Bus Selector3 : BusSelector  OutputSignals=Translation_States.VEL_u_K_R_E_B_mDs,Translation_States.VEL_v_K_R_E_B_mDs,Translation_States.VEL_w_K_R_E_B_mDs
  Bus Selector4 : BusSelector  OutputSignals=Attitude_States
  Bus Selector5 : BusSelector  OutputSignals=Attitude_States.ATT_Phi_rad
  Bus Selector6 : BusSelector  OutputSignals=Attitude_States
  Bus Selector7 : BusSelector  OutputSignals=Position_States.POS_WGS84.POS_mue_ WGS84_rad,Position_States.POS_WGS84.POS_h_ WGS84_m
  Bus Selector8 : BusSelector  OutputSignals=Attitude_States.ATT_Phi_rad,Attitude_States.ATT_Theta_rad,Attitude_States.ATT_Psi_rad
  Bus Selector9 : BusSelector  OutputSignals=FDM_Ctrl.enable_gravity_flg
  Constant3 : Constant  Value=-1
  Divide : Product  Inputs=*/
  Drag : Subsystem  TreatAsAtomicUnit=on
  Gravity : Subsystem  TreatAsAtomicUnit=on
  NED2PosWGS84Dot : Subsystem
  Propulsion : Subsystem
  Reverse Fin Deflection : lib_Fin_Deflections/Reverse Fin Deflection  Control_Surfaces=HIL_Data.Control_Surfaces
  dp2az : TransferFcn  Numerator=TF.dp2az.num  Denominator=TF.dp2az.denom
  dp2pitch : TransferFcn  Numerator=TF.dp2pitch.num  Denominator=TF.dp2pitch.denom
  dr2roll : TransferFcn  Numerator=TF.dr2roll.num  Denominator=TF.dr2roll.denom
  dy2ay : TransferFcn  Numerator=TF.dy2ay.num  Denominator=TF.dy2ay.denom
  dy2yaw : TransferFcn  Numerator=TF.dy2yaw.num  Denominator=TF.dy2yaw.denom
  pqr2EulerDot : Subsystem
  uvw2PosNEDDot : Subsystem
  FDM_states : Outport  OutDataTypeStr=Bus: FDM_States_Bus  VectorParamsAs1DForOutWhenUnconnected=off
  FDM_Rot_Body : Outport  Port=2  OutDataTypeStr=Bus: FDM_Rot_Body_Bus  VectorParamsAs1DForOutWhenUnconnected=off
  FDM_States_Dot : Outport  Port=3  OutDataTypeStr=Bus: FDM_States_Dot_Bus  VectorParamsAs1DForOutWhenUnconnected=off
  wires:
  Reverse Fin Deflection/3 -> dy2yaw/1, dy2ay/1  "delta_y"
  Bus Selector2/1 -> Propulsion/Enable  "<enable_propulsion_flg>"
  dr2roll/1 -> pqr2EulerDot/2(p), Bus Creator7/1  "p_B_radDs"
  dp2pitch/1 -> pqr2EulerDot/3(q), Bus Creator7/2  "q_B_radDs"
  Reverse Fin Deflection/2 -> dp2pitch/1, dp2az/1  "delta_p"
  Reverse Fin Deflection/1 -> dr2roll/1  "delta_r"
  dy2yaw/1 -> Bus Creator7/3, pqr2EulerDot/4(r)  "r_B_radDs"
  Propulsion/1(F_x_prop_N) -> Divide/1
  Bus Creator/1 -> FDM_States_Dot/1
  pqr2EulerDot/3(psi_dot) -> Bus Creator1/3  "ATT_Dot_Psi_radDs"
  pqr2EulerDot/2(theta_dot) -> Bus Creator1/2  "ATT_Dot_Theta_radDs"
  pqr2EulerDot/1(phi_dot) -> Bus Creator1/1  "ATT_Dot_Phi_radDs"
  Bus Creator1/1 -> Bus Creator/1  "ATT_Euler_Dot"
  Bus Creator2/1 -> Bus Creator/2  "Translation_States_Dot"
  dp2az/1 -> Add2/1
  dy2ay/1 -> Add1/1
  Divide/1 -> Add/1
  Add/1 -> Bus Creator2/1  "ACC_x_B_mDs2"
  Add1/1 -> Bus Creator2/2  "ACC_y_B_mDs2"
  Add2/1 -> Bus Creator2/3  "ACC_z_B_mDs2"
  NED2PosWGS84Dot/3(h_dot_mDs) -> Bus Creator3/3  "POS_h_Dot_WGS84_mDs"
  NED2PosWGS84Dot/2(mue_dot_radDs) -> Bus Creator3/2  "POS_mue_Dot_WGS84_radDs"
  NED2PosWGS84Dot/1(lambda_dot_radDs) -> Bus Creator3/1  "POS_lambda_Dot_WGS84_radDs"
  Bus Creator4/1 -> Bus Creator/4  "Airframe_States_Dot"
  Propulsion/2(motor_state_perc_dot) -> Bus Creator4/1  "Motor_state_dot_percDs"
  External_Inputs/1 -> Bus Selector1/1
  Simulation_Control/1 -> Bus Selector10/1, Bus Selector9/1, Bus Selector2/1
  Bus Selector1/1 -> Propulsion/1(Motor_Ignition_flg)  "<Motor_Ignition_flg>"
  Bus Selector4/1 -> pqr2EulerDot/1(ATT)  "<Attitude_States>"
  Bus Selector5/1 -> Reverse Fin Deflection/1  "<ATT_Phi_rad>"
  Control_Surface_Deflections/1 -> Reverse Fin Deflection/2
  Bus Selector/1 -> Divide/2  "<mass_kg>"
  Bus Selector3/1 -> uvw2PosNEDDot/1(u)  "<VEL_u_K_R_E_B_mDs>"
  Bus Selector3/2 -> uvw2PosNEDDot/2(v)  "<VEL_v_K_R_E_B_mDs>"
  Bus Selector3/3 -> uvw2PosNEDDot/3(w)  "<VEL_w_K_R_E_B_mDs>"
  uvw2PosNEDDot/1(x_dot_mDs) -> Bus Creator5/1, NED2PosWGS84Dot/3(x_dot_NED_mDs)  "POS_x_Dot_NED_mDs"
  uvw2PosNEDDot/2(y_dot_mDs) -> NED2PosWGS84Dot/4(y_dot_NED_mDs), Bus Creator5/2  "POS_y_Dot_NED_mDs"
  uvw2PosNEDDot/3(z_dot_mDs) -> NED2PosWGS84Dot/5(z_dot_NED_mDs), Bus Creator5/3  "POS_z_Dot_NED_mDs"
  Bus Creator6/1 -> Bus Creator/3  "Position_States_Dot"
  Bus Creator3/1 -> Bus Creator6/1  "POS_WGS84_Dot"
  Bus Creator5/1 -> Bus Creator6/2  "POS_NED_Dot"
  Bus Selector6/1 -> uvw2PosNEDDot/4(ATT)  "<Attitude_States>"
  Bus Selector7/1 -> NED2PosWGS84Dot/1(mue_rad)  "<POS_mue_ WGS84_rad>"
  Bus Selector7/2 -> NED2PosWGS84Dot/2(h_m)  "<POS_h_ WGS84_m>"
  Gravity/1(acc_x_grav_mDs) -> Add/2
  Constant3/1 -> Drag/2(beta), Drag/1(alpha)
  Gravity/2(acc_y_grav_mDs) -> Add1/2
  Gravity/3(acc_z_grav_mDs) -> Add2/2
  Bus Selector8/1 -> Gravity/1(phi)  "<ATT_Phi_rad>"
  Bus Selector8/2 -> Gravity/2(theta)  "<ATT_Theta_rad>"
  Bus Selector8/3 -> Gravity/3(psi)  "<ATT_Psi_rad>"
  Bus Selector9/1 -> Gravity/Enable  "<enable_gravity_flg>"
  Bus Selector10/1 -> Drag/Enable  "<enable_drag_flg>"
  Drag/1(acc_x_drag_mDs2) -> Add/3
  Drag/2(acc_y_drag_mDs2) -> Add1/3
  Drag/3(acc_z_drag_mDs2) -> Add2/3
  FDM_States/1 -> FDM_states/1, Bus Selector5/1, Bus Selector6/1, Bus Selector3/1, Bus Selector7/1, Bus Selector8/1, Bus Selector/1, Bus Selector4/1
  Bus Creator7/1 -> FDM_Rot_Body/1
